simulink library "House_simple"  (R2018b)
settings: Solver=ode45  StartTime=0.0  StopTime=10.0  RelTol=1e-3  EnableMultiTasking=on
undefined symbols (not defined in the file): path_carnot
libraries: carnot x4, simulink_extras x3
settings Model: Creator=bernd.hafner  LastModifiedBy=P41573
settings DataIOCC: LimitDataPoints=on  SaveFormat=Array  SignalLoggingSaveFormat=ModelDataLogs
settings OptimizationCC: ExpressionDepthLimit=2147483647  LifeSpan=inf
settings DebuggingCC: UnderspecifiedInitializationDetection=Classic  MergeDetectMultiDrivingBlocksExec=none  SolverPrmCheckMsg=warning  FcnCallInpInsideContextMsg=warning  StateNameClashWarn=warning  SFUnexpectedBacktrackingDiag=warning  SFNoUnconditionalDefaultTransitionDiag=warning  SFExecutionAtInitializationDiag=none
settings HardwareCC: ProdBitPerPointer=32  ProdBitPerSizeT=32  ProdBitPerPtrDiffT=32  ProdLargestAtomicFloat=None  ProdIntDivRoundTo=Undefined  ProdEndianess=Unspecified  ProdWordSize=32  ProdHWDeviceType=32-bit Generic
settings ModelReferenceCC: PropagateSignalLabelsOutOfModel=off
settings SFSimCC: SimUseLocalCustomCode=off
settings RTWCC: RTWUseLocalCustomCode=off
settings CodeAppCC: StateflowObjectComments=on
settings GRTTargetCC: TargetLangStandard=C89/C90 (ANSI)  GeneratePreprocessorConditionals=Disable all  CombineOutputUpdateFcns=off  GRTInterface=on
settings ConfigComp: CovMetricSettings=dw  CovHtmlReporting=on  CovSaveCumulativeToWorkspaceVar=on  CovSaveSingleToWorkspaceVar=on  CovExternalEMLEnable=off

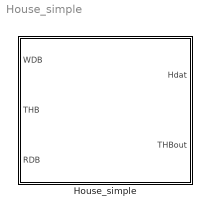
== system House_simple ==
  House_simple : Subsystem  mask(House simple){tini=20, dtroom=inf, Tmeaninside=23.8, deltathetai=3.8, Tmeanoutside=11, deltathetae=9.3, tshift=319*3600, PathName=fullfile(path_carnot('libsl'), 'Load', 'Houses', 'House_simple', 'parameter_set'), FileName='Default_SimpleHouseISOgm.mat', userPath=off, userParam=off, Ahabit=140, Hroom=2.5, slabwidth=10, slablength=7, dwall=0.4, UAwall=100, capa=500000, utot=0.183, gammat=0, cond_ground=2, cp_ground=800, rho_ground=2500, Awindow=[12 4 3 4], AziWin=[0 90 -180 -90], Uwindow=[2 2 2 2], Gwindow=[0.5 0.5 0.5 0.5], alpha=10, H=1.2, W=1, Nwin=4, Ventilationrate=0.4, Heatrecovery=0, pnom=10000, dtnom=49.83, expo=1.3, mcap=10*4812, lin=100, qua=100}
      mask prompts: tini "Initial temperature in °C"; dtroom "Max. change of room temperature in K (standard value is 'inf')"; Tmeaninside "Mean inside temperature over one year [°C]"; deltathetai "Amplitude of monthly mean inside temperature over the year [K]"; Tmeanoutside "Mean outside temperature over one year [°C]"; deltathetae "Amplitude of monthly mean outside temperature over the year [K]"; tshift "Time shift where outside temperature sine-curve shows a mimimum [s]"; PathName "Path"; FileName "Parameter set"; userPath "Edit path and name of parameter set"; userParam "User defined parameters"; Ahabit "Heated living surface in m²"; Hroom "Height of rooms in m"; slabwidth "Width of slab in m"; slablength "Length of slab in m"; dwall "Average thickness of walls inlcuding insulation [m]"; UAwall "Total heat transfer to ambient (walls/roof) in W/K"; capa "Thermal capactiy per surface in J/m²/K"; utot "Total heat transfer of slab to ground [W/m²/K]"; gammat "linear thermal transmittance associated with wall/floor junctions [W/mK]"; cond_ground "conductivity of ground [W/(m*K)]"; cp_ground "capacity of ground [J/(kg*K)]"; rho_ground "density of ground [kg/m^3]"; Awindow "Surface of 4 windows in m² (vector)"; AziWin "Orientation of the 4 windows (south 0, east -90,west 90)"; Uwindow "Heat loss coefficient 4 windows in W/m²/K [vector]"; Gwindow "Light transmittance 4 windows (0..1) * (1 - frame_part) [vector]"; alpha "Maximal opening angle in °"; H "Height of window opening in m"; W "Width of window opening in m"; Nwin "Number of windows for ventilation"; Ventilationrate "Ventilation rate in 1/h"; Heatrecovery "Heat recovery (0..1)"; pnom "Qdot_nom: nominal power in W"; dtnom "Tdiff_nom: nominal temperature difference in K"; expo "Radiator exponent (> 0)"; mcap "mass * capacity in J/K"; lin "l : linear pressure drop Pa/(kg/s)"; qua "q : quadratic pressure drop Pa/(kg/s)²"
      mask help:
      | Simple model of a house with one thermal node. The geometry is a box with a flat roof and 4 windows (see House_OneNodeModel). The heat transfer to the ground is modeled by HeatTransfer2Ground_ISO13370. The heating system is the Radiator model. The ventilation an heat recovery uses the Ventilation model. Resident data like internal gains, window opening and shading are defined by the Resident Data Bus RDB.
      |
      | Max. change of room temperatue: Set parameter to 0 K to calculate idealized heating behaviour. The power balance (Qdot_all) is the theoretical heating demand (see example_House_Ideal.slx).
      mask init:
      | [ok, param] = CarnotCallbacks_HouseSimple('SetParameters',gcbh,PathName,FileName);
      mask Help: web(fullfile(path_carnot('help'),'houseSimple.html'),'-helpbrowser')
      mask TypeOptions tini: House_OneNodeModel/tini | Radiator/tini
      mask TypeOptions dtroom: House_OneNodeModel/dtroom
      mask TypeOptions Tmeaninside: HeatTransfer2Ground_ISO13370/Tmeaninside
      mask TypeOptions deltathetai: HeatTransfer2Ground_ISO13370/deltathetai
      mask TypeOptions Tmeanoutside: HeatTransfer2Ground_ISO13370/Tmeanoutside
      mask TypeOptions deltathetae: HeatTransfer2Ground_ISO13370/deltathetae
      mask TypeOptions tshift: HeatTransfer2Ground_ISO13370/tshift
      mask Callback userPath: [ok, param] = CarnotCallbacks_HouseSimple('UserEdit',gcbh);
      mask Callback userParam: [ok, param] = CarnotCallbacks_HouseSimple('UserEdit',gcbh);
      mask TypeOptions Ahabit: House_OneNodeModel/A | Ventilation/Ahabit | Ahabit/Value
      mask TypeOptions Hroom: Simple_House_ISO_GroundModel/Hroom | Ventilation/Hroom
      mask TypeOptions slabwidth: HeatTransfer2Ground_ISO13370/slabwidth
      mask TypeOptions slablength: HeatTransfer2Ground_ISO13370/slablength
      mask TypeOptions dwall: HeatTransfer2Ground_ISO13370/dwall
      mask TypeOptions UAwall: House_OneNodeModel/UAout
      mask TypeOptions capa: House_OneNodeModel/capa
      mask TypeOptions utot: HeatTransfer2Ground_ISO13370/utot
      mask TypeOptions gammat: HeatTransfer2Ground_ISO13370/gammat
      mask TypeOptions cond_ground: HeatTransfer2Ground_ISO13370/cond_ground
      mask TypeOptions cp_ground: HeatTransfer2Ground_ISO13370/cp_ground
      mask TypeOptions rho_ground: HeatTransfer2Ground_ISO13370/rho_ground
      mask TypeOptions Awindow: House_OneNodeModel/Awin
      mask TypeOptions AziWin: House_OneNodeModel/AziWin
      mask TypeOptions Uwindow: House_OneNodeModel/Uwin
      mask TypeOptions Gwindow: House_OneNodeModel/Gwin
      mask TypeOptions alpha: Ventilation/alpha
      mask TypeOptions H: Ventilation/H
      mask TypeOptions W: Ventilation/W
      mask TypeOptions Nwin: Ventilation/Nwin
      mask TypeOptions Ventilationrate: Ventilation/vent
      mask TypeOptions Heatrecovery: Ventilation/rec
      mask TypeOptions pnom: Radiator/pnom
      mask TypeOptions dtnom: Radiator/dtnom
      mask TypeOptions expo: Radiator/expo
      mask TypeOptions mcap: Radiator/mcap
      mask TypeOptions lin: Radiator/lin
      mask TypeOptions qua: Radiator/qua
      mask DialogControl Container10 Prompt: Calculation
      mask DialogControl ParameterGroupFile Prompt: Picking a parameter set
      mask DialogControl Control1 Prompt: Carnot public data
      mask DialogControl Control1 Callback: [ok, file] = CarnotCallbacks_HouseSimple('GetFilename',gcbh, 'public');
      mask DialogControl Control3 Prompt: Carnot internal data
      mask DialogControl Control3 Callback: [ok, file] = CarnotCallbacks_HouseSimple('GetFilename',gcbh, 'internal');
      mask DialogControl Control4 Prompt: Selected path
      mask DialogControl Control4 Callback: [ok, file] = CarnotCallbacks_HouseSimple('GetFilename',gcbh, 'selected');
      mask DialogControl Container5 Prompt: House
      mask DialogControl Container13 Prompt: Ground
      mask DialogControl Container8 Prompt: Windows
      mask DialogControl Container9 Prompt: HVAC
      mask DialogControl Control5 Prompt: Save in Carnot internal data
      mask DialogControl Control5 Callback: [ok, param] = CarnotCallbacks_HouseSimple('SaveFilename',gcbh, 'internal','SH');
      mask DialogControl Control6 Prompt: Save in selected path
      mask DialogControl Control6 Callback: [ok, param] = CarnotCallbacks_HouseSimple('SaveFilename',gcbh, 'selected','SH');
      mask Display:
      | % user defined picture file
      | picfile = fullfile(path_carnot('intlibsl'), ...
      |         'Load','Houses','Simple_House_ISOgm_CONF','parameter_set', ...
      |         'Simple_House_ISOgm_CONF.jpg');
      | 
      | % show internal picture if defined
      | if ~BlockIsInCarnotLibrary ...      % if not located in library any more
      |         && exist(picfile,'file')    % AND picfile is present
      |     image(imread(picfile), [0.15 0.1 0.7 0.8])
      |     set_param(gcb, 'BackgroundColor', 'White')
      | else
      |     % show public picture
      |     plot([10,10,90,90,10]/120+0.1, [0,50,50,0,0]/100+0.1,...
      |          [100,60,40,0]/120+0.1,    [40,80,80,40]/100+0.1,...
      |          [20,34,34,20,20]/120+0.1, [40,40,20,20,40]/100+0.1,...
      |          [60,60,40,40]/120+0.1,    [0,40,40,0]/100+0.1,...
      |          [65,80,80,65,65]/120+0.1, [40,40,20,20,40]/100+0.1,...
      |          [47,54,54,47,47]/120+0.1, [35,35,4,4,35]/100+0.1,...
      |          [45,41]/120+0.1,          [20,20]/100+0.1)
      |      set_param(gcb, 'BackgroundColor', 'Orange')
      | end

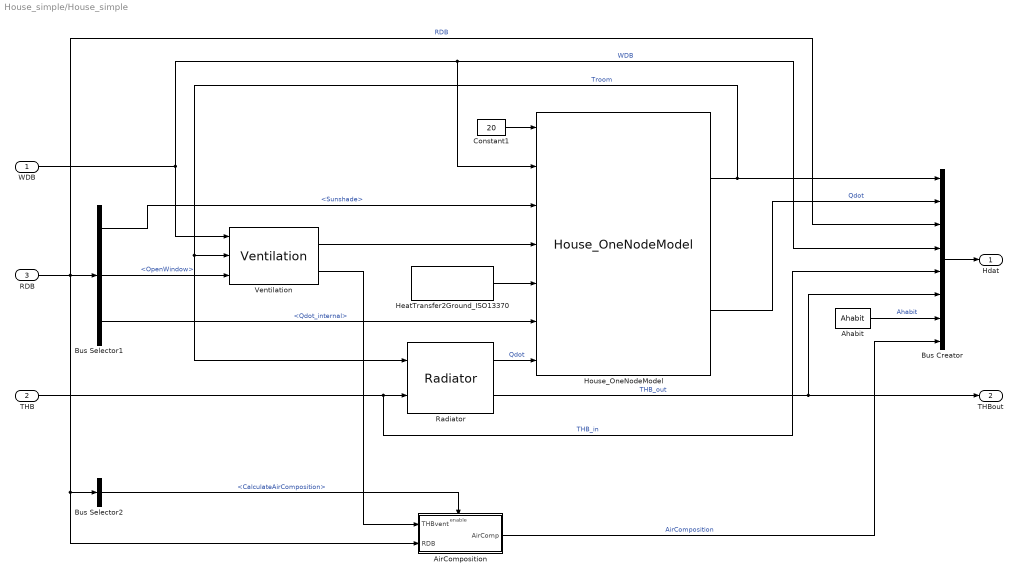
== system House_simple/House_simple ==
  WDB : Inport
  THB : Inport  Port=2
  RDB : Inport  Port=3
  Ahabit : Constant  Value=Ahabit
  AirComposition : Subsystem
  Bus Creator : BusCreator  Inputs=8
  Bus Selector1 : BusSelector  OutputSignals=Sunshade,OpenWindow,Qdot_internal
  Bus Selector2 : BusSelector  OutputSignals=CalculateAirComposition
  Constant1 : Constant  Value=20
  HeatTransfer2Ground_ISO13370 : carnot/Basic/Heat_Transfer/HeatTransfer2Ground_ISO13370  slabwidth=slabwidth  slablength=slablength  gammat=gammat  Tmeaninside=Tmeaninside  deltathetai=deltathetai  Tmeanoutside=Tmeanoutside  deltathetae=deltathetae  tshift=tshift  dwall=dwall  cond_ground=cond_ground  cp_ground=cp_ground  rho_ground=rho_ground  utot=utot
      settings: SourceProductName=Carnot
  House_OneNodeModel : carnot/Basic/Thermal_Models/House_OneNodeModel  A=Ahabit  UAout=UAwall  UAin=0  capa=capa  tini=tini  dtroom=dtroom  AziWin=AziWin  Awin=Awindow  Uwin=Uwindow  Gwin=Gwindow
      settings: SourceProductName=Carnot
  Radiator : carnot/Source/Heat_Exchanger/Radiator  pnom=pnom  dtnom=dtnom  expo=expo  mcap=mcap  tini=tini  lin=lin  qua=qua
      settings: SourceProductName=Carnot
  Ventilation : carnot/Source/Ventilation/Ventilation  Ahabit=Ahabit  Hroom=Hroom  vent=Ventilationrate  rec=Heatrecovery  ppmCO2=400  ppmVOC=0  alpha=alpha  H=H  W=W  Nwin=Nwin
      settings: SourceProductName=Carnot
  Hdat : Outport
  THBout : Outport  Port=2
  wires:
  Bus Selector1/2 -> Ventilation/3  "<OpenWindow>"
  Bus Selector1/1 -> House_OneNodeModel/3  "<Sunshade>"
  RDB/1 -> Bus Creator/3, AirComposition/2(RDB), Bus Selector2/1, Bus Selector1/1  "RDB"
  WDB/1 -> Bus Creator/4, House_OneNodeModel/2, Ventilation/1  "WDB"
  Ventilation/1 -> House_OneNodeModel/4
  Radiator/1 -> House_OneNodeModel/7  "Qdot"
  Bus Selector1/3 -> House_OneNodeModel/6  "<Qdot_internal>"
  Constant1/1 -> House_OneNodeModel/1
  HeatTransfer2Ground_ISO13370/1 -> House_OneNodeModel/5
  Bus Creator/1 -> Hdat/1
  House_OneNodeModel/2 -> Bus Creator/2  "Qdot"
  House_OneNodeModel/1 -> Bus Creator/1, Radiator/1, Ventilation/2  "Troom"
  Radiator/2 -> Bus Creator/6, THBout/1  "THB_out"
  THB/1 -> Bus Creator/5, Radiator/2  "THB_in"
  Ahabit/1 -> Bus Creator/7  "Ahabit"
  Bus Selector2/1 -> AirComposition/Enable  "<CalculateAirComposition>"
  AirComposition/1(AirComp) -> Bus Creator/8  "AirComposition"
  Ventilation/2 -> AirComposition/1(THBvent)

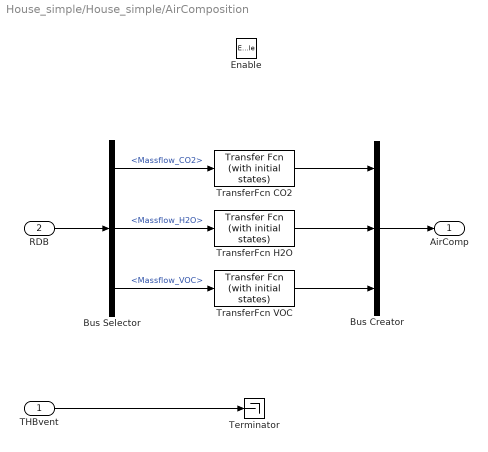
== system House_simple/House_simple/AirComposition ==
  THBvent : Inport
  RDB : Inport  Port=2
  Enable : EnablePort
  Bus Creator : BusCreator  Inputs=3
  Bus Selector : BusSelector  OutputSignals=Massflow_CO2,Massflow_H2O,Massflow_VOC
  Terminator : Terminator
  TransferFcn CO2 : simulink_extras/Additional Linear/Transfer Fcn (with initial states)  N=[1]  D="[1  1]"  X0=.5
  TransferFcn H2O : simulink_extras/Additional Linear/Transfer Fcn (with initial states)  N=[1]  D="[1  1]"  X0=.5
  TransferFcn VOC : simulink_extras/Additional Linear/Transfer Fcn (with initial states)  N=[1]  D="[1  1]"  X0=.5
  AirComp : Outport
  wires:
  RDB/1 -> Bus Selector/1
  Bus Selector/1 -> TransferFcn CO2/1  "<Massflow_CO2>"
  Bus Selector/3 -> TransferFcn VOC/1  "<Massflow_VOC>"
  Bus Selector/2 -> TransferFcn H2O/1  "<Massflow_H2O>"
  Bus Creator/1 -> AirComp/1
  TransferFcn CO2/1 -> Bus Creator/1
  TransferFcn H2O/1 -> Bus Creator/2
  TransferFcn VOC/1 -> Bus Creator/3
  THBvent/1 -> Terminator/1
